simulink model "model"  (R2018a)
settings: Solver=VariableStepAuto  StartTime=0.0  StopTime=10.0  RelTol=1e-3
settings Model: Creator=Rafael  LastModifiedBy=Rafael

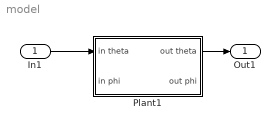
== system model ==
  In1 : Inport
  Plant1 : Subsystem
  Out1 : Outport
  wires:
  Plant1/1(out theta) -> Out1/1
  In1/1 -> Plant1/1(in theta)

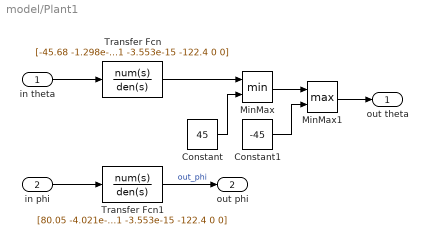
== system model/Plant1 ==
  in theta : Inport
  in phi : Inport  Port=2
  Constant : Constant  Value=45
  Constant1 : Constant  Value=-45
  MinMax : MinMax  Inputs=2
  MinMax1 : MinMax  Function=max  Inputs=2
  Transfer Fcn : TransferFcn  Numerator=[-45.68 -1.298e-11 7.179e-13]  Denominator=[1 -3.553e-15 -122.4 0 0]
  Transfer Fcn1 : TransferFcn  Numerator=[80.05 -4.021e-12 61140]  Denominator=[1 -3.553e-15 -122.4 0 0]
  out theta : Outport
  out phi : Outport  Port=2
  wires:
  Transfer Fcn1/1 -> out phi/1  "out_phi"
  in theta/1 -> Transfer Fcn/1
  in phi/1 -> Transfer Fcn1/1
  MinMax1/1 -> out theta/1
  Transfer Fcn/1 -> MinMax/1
  Constant/1 -> MinMax/2
  Constant1/1 -> MinMax1/2
  MinMax/1 -> MinMax1/1
